simulink model "ModelanfisD1"  (R2017a)
settings: Solver=VariableStepAuto  StartTime=0.0  StopTime=578  RelTol=1e-3
values from neighbouring files (symbols this model uses):
  dinnegc12 = [-0.01 -0.01 -0.02 -0.01 -0.01 -0.01 0 0 0 0 0.01 -0.01 ... (2312 elements, 578x4)]    [anfisd.mat]    (also in anfisfin.mat; cinco.mat)
libraries: dspsrcs4 x84, fuzblock x24
settings Model: Creator=Dell  LastModifiedBy=Dell

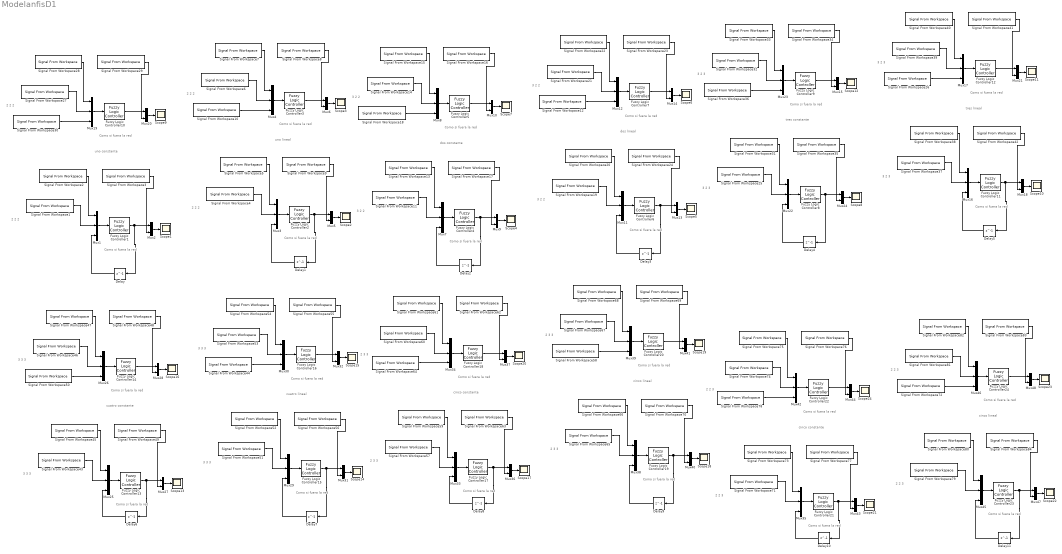
== system ModelanfisD1 ==
  note: 2 2 2
  note: Como si fuera la red
  note: uno constante
  note: 2 2 2
  note: Como si fuera la red
  note: 2 2 2
  note: Como si fuera la red
  note: uno lineal
  note: 2 2 2
  note: Como si fuera la red
  note: 3 2 2
  note: Como si fuera la red
  note: dos constante
  note: 3 2 2
  note: Como si fuera la red
  note: 3 2 2
  note: Como si fuera la red
  note: dos lineal
  note: 3 2 2
  note: Como si fuera la red
  note: 3 2 3
  note: Como si fuera la red
  note: tres constante
  note: 3 2 3
  note: 3 2 3
  note: Como si fuera la red
  note: tres lineal
  note: 3 2 3
  note: Como si fuera la red
  note: 3 3 3
  note: Como si fuera la red
  note: cuatro constante
  note: 3 3 3
  note: Como si fuera la red
  note: 3 3 3
  note: Como si fuera la red
  note: cuatro lineal
  note: 3 3 3
  note: Como si fuera la red
  note: 2 3 3
  note: Como si fuera la red
  note: cinco constante
  note: 2 3 3
  note: Como si fuera la red
  note: 2 3 3
  note: Como si fuera la red
  note: cinco lineal
  note: 2 3 3
  note: Como si fuera la red
  note: 2 2 3
  note: Como si fuera la red
  note: cinco constante
  note: 2 2 3
  note: Como si fuera la red
  note: 2 2 3
  note: Como si fuera la red
  note: cinco lineal
  note: 2 2 3
  note: Como si fuera la red
  Delay{,1..11} (12 alike) : Delay  DelayLength=1  InitialCondition=0
  Fuzzy Logic Controller1 : fuzblock/Fuzzy Logic  Controller  fis=uno
  Fuzzy Logic Controller10 : fuzblock/Fuzzy Logic  Controller  fis=uno
  Fuzzy Logic Controller11 : fuzblock/Fuzzy Logic  Controller  fis=tres3
  Fuzzy Logic Controller12 : fuzblock/Fuzzy Logic  Controller  fis=tres3
  Fuzzy Logic Controller13 : fuzblock/Fuzzy Logic  Controller  fis=cuatro
  Fuzzy Logic Controller14 : fuzblock/Fuzzy Logic  Controller  fis=cuatro
  Fuzzy Logic Controller15 : fuzblock/Fuzzy Logic  Controller  fis=cuatro4
  Fuzzy Logic Controller16 : fuzblock/Fuzzy Logic  Controller  fis=cuatro4
  Fuzzy Logic Controller17 : fuzblock/Fuzzy Logic  Controller  fis=cinco
  Fuzzy Logic Controller18 : fuzblock/Fuzzy Logic  Controller  fis=cinco
  Fuzzy Logic Controller19 : fuzblock/Fuzzy Logic  Controller  fis=cinco5
  Fuzzy Logic Controller2 : fuzblock/Fuzzy Logic  Controller  fis=Uno1
  Fuzzy Logic Controller20 : fuzblock/Fuzzy Logic  Controller  fis=cinco5
  Fuzzy Logic Controller21 : fuzblock/Fuzzy Logic  Controller  fis=seis
  Fuzzy Logic Controller22 : fuzblock/Fuzzy Logic  Controller  fis=seis
  Fuzzy Logic Controller23 : fuzblock/Fuzzy Logic  Controller  fis=seis6
  Fuzzy Logic Controller24 : fuzblock/Fuzzy Logic  Controller  fis=seis6
  Fuzzy Logic Controller3 : fuzblock/Fuzzy Logic  Controller  fis=Uno1
  Fuzzy Logic Controller4 : fuzblock/Fuzzy Logic  Controller  fis=dos
  Fuzzy Logic Controller5 : fuzblock/Fuzzy Logic  Controller  fis=dos
  Fuzzy Logic Controller6 : fuzblock/Fuzzy Logic  Controller  fis=dos2
  Fuzzy Logic Controller7 : fuzblock/Fuzzy Logic  Controller  fis=dos2
  Fuzzy Logic Controller8 : fuzblock/Fuzzy Logic  Controller  fis=tres
  Fuzzy Logic Controller9 : fuzblock/Fuzzy Logic  Controller  fis=tres
  Mux{1,3..4,7..8,11..12,16..17,19,22..23,25..26,29..30,33..35,38..39,42,45..46} (24 alike) : Mux  Inputs=3
  Mux{2,5..6,9..10,13..15,18,20..21,24,27..28,31..32,36..37,40..41,43..44,47..48} (24 alike) : Mux  Inputs=2
  Scope{1..24} (24 alike) : Scope
  Signal From Workspace{1,4,6,11,14,19,21,25,27,32,37,39,43,46,51,53,57,60,65,67,71,74,79,81} (24 alike) : dspsrcs4/Signal From Workspace  X=dinnegc12(:,2)  Ts=1  nsamps=1  OutputAfterFinalValue=Setting to zero  ignoreOrWarnInputAndFrameLengths=off  OutputFrames=off
  Signal From Workspace{10,12,18,26,30,36,44,50,58,64,72,78} (12 alike) : dspsrcs4/Signal From Workspace  X=dinnegc12(:,3)  Ts=1  nsamps=1  OutputAfterFinalValue=Setting to zero  ignoreOrWarnInputAndFrameLengths=off  OutputFrames=off
  Signal From Workspace{2,5,7,13,15,20,22,28,31,33,38,40,45,47,52,54,59,61,66,68,73,75,80,82} (24 alike) : dspsrcs4/Signal From Workspace  X=dinnegc12(:,1)  Ts=1  nsamps=1  OutputAfterFinalValue=Setting to zero  ignoreOrWarnInputAndFrameLengths=off  OutputFrames=off
  Signal From Workspace{3,8..9,16..17,23..24,29,34..35,41..42,48..49,55..56,62..63,69..70,76..77,83..84} (24 alike) : dspsrcs4/Signal From Workspace  X=dinnegc12(:,4)  Ts=1  nsamps=1  OutputAfterFinalValue=Setting to zero  ignoreOrWarnInputAndFrameLengths=off  OutputFrames=off
  wires:
  Signal From Workspace30/1 -> Mux19/3
  Signal From Workspace27/1 -> Mux19/2
  Fuzzy Logic Controller10/1 -> Mux20/1
  Signal From Workspace28/1 -> Mux19/1
  Mux20/1 -> Scope9/1
  Signal From Workspace29/1 -> Mux20/2
  Mux19/1 -> Fuzzy Logic Controller10/1
  Mux1/1 -> Fuzzy Logic Controller1/1
  Signal From Workspace3/1 -> Mux2/2
  Mux2/1 -> Scope1/1
  Signal From Workspace2/1 -> Mux1/1
  Fuzzy Logic Controller1/1 -> Delay/1, Mux2/1
  Signal From Workspace1/1 -> Mux1/2
  Delay/1 -> Mux1/3
  Delay1/1 -> Mux3/3
  Signal From Workspace4/1 -> Mux3/2
  Fuzzy Logic Controller2/1 -> Mux5/1, Delay1/1
  Signal From Workspace5/1 -> Mux3/1
  Mux5/1 -> Scope2/1
  Signal From Workspace9/1 -> Mux5/2
  Mux3/1 -> Fuzzy Logic Controller2/1
  Mux4/1 -> Fuzzy Logic Controller3/1
  Signal From Workspace8/1 -> Mux6/2
  Mux6/1 -> Scope3/1
  Signal From Workspace7/1 -> Mux4/1
  Fuzzy Logic Controller3/1 -> Mux6/1
  Signal From Workspace6/1 -> Mux4/2
  Signal From Workspace10/1 -> Mux4/3
  Signal From Workspace12/1 -> Mux12/3
  Signal From Workspace21/1 -> Mux12/2
  Fuzzy Logic Controller7/1 -> Mux14/1
  Signal From Workspace22/1 -> Mux12/1
  Mux14/1 -> Scope6/1
  Signal From Workspace23/1 -> Mux14/2
  Mux12/1 -> Fuzzy Logic Controller7/1
  Mux11/1 -> Fuzzy Logic Controller6/1
  Signal From Workspace24/1 -> Mux13/2
  Mux13/1 -> Scope5/1
  Signal From Workspace20/1 -> Mux11/1
  Fuzzy Logic Controller6/1 -> Delay3/1, Mux13/1
  Signal From Workspace19/1 -> Mux11/2
  Delay3/1 -> Mux11/3
  Delay2/1 -> Mux7/3
  Signal From Workspace11/1 -> Mux7/2
  Fuzzy Logic Controller4/1 -> Mux9/1, Delay2/1
  Signal From Workspace13/1 -> Mux7/1
  Mux9/1 -> Scope4/1
  Signal From Workspace17/1 -> Mux9/2
  Mux7/1 -> Fuzzy Logic Controller4/1
  Mux8/1 -> Fuzzy Logic Controller5/1
  Signal From Workspace16/1 -> Mux10/2
  Mux10/1 -> Scope7/1
  Signal From Workspace15/1 -> Mux8/1
  Fuzzy Logic Controller5/1 -> Mux10/1
  Signal From Workspace14/1 -> Mux8/2
  Signal From Workspace18/1 -> Mux8/3
  Signal From Workspace36/1 -> Mux23/3
  Signal From Workspace32/1 -> Mux23/2
  Fuzzy Logic Controller9/1 -> Mux15/1
  Signal From Workspace33/1 -> Mux23/1
  Mux15/1 -> Scope12/1
  Signal From Workspace34/1 -> Mux15/2
  Mux23/1 -> Fuzzy Logic Controller9/1
  Mux22/1 -> Fuzzy Logic Controller8/1
  Signal From Workspace35/1 -> Mux24/2
  Mux24/1 -> Scope8/1
  Signal From Workspace31/1 -> Mux22/1
  Fuzzy Logic Controller8/1 -> Delay4/1, Mux24/1
  Signal From Workspace25/1 -> Mux22/2
  Delay4/1 -> Mux22/3
  Delay5/1 -> Mux16/3
  Signal From Workspace37/1 -> Mux16/2
  Fuzzy Logic Controller11/1 -> Delay5/1, Mux18/1
  Signal From Workspace38/1 -> Mux16/1
  Mux18/1 -> Scope10/1
  Signal From Workspace42/1 -> Mux18/2
  Mux16/1 -> Fuzzy Logic Controller11/1
  Mux17/1 -> Fuzzy Logic Controller12/1
  Signal From Workspace41/1 -> Mux21/2
  Mux21/1 -> Scope11/1
  Signal From Workspace40/1 -> Mux17/1
  Fuzzy Logic Controller12/1 -> Mux21/1
  Signal From Workspace39/1 -> Mux17/2
  Signal From Workspace26/1 -> Mux17/3
  Signal From Workspace44/1 -> Mux30/3
  Signal From Workspace53/1 -> Mux30/2
  Fuzzy Logic Controller16/1 -> Mux32/1
  Signal From Workspace54/1 -> Mux30/1
  Mux32/1 -> Scope15/1
  Signal From Workspace55/1 -> Mux32/2
  Mux30/1 -> Fuzzy Logic Controller16/1
  Mux29/1 -> Fuzzy Logic Controller15/1
  Signal From Workspace56/1 -> Mux31/2
  Mux31/1 -> Scope14/1
  Signal From Workspace52/1 -> Mux29/1
  Fuzzy Logic Controller15/1 -> Delay7/1, Mux31/1
  Signal From Workspace51/1 -> Mux29/2
  Delay7/1 -> Mux29/3
  Delay6/1 -> Mux25/3
  Signal From Workspace43/1 -> Mux25/2
  Fuzzy Logic Controller13/1 -> Mux27/1, Delay6/1
  Signal From Workspace45/1 -> Mux25/1
  Mux27/1 -> Scope13/1
  Signal From Workspace49/1 -> Mux27/2
  Mux25/1 -> Fuzzy Logic Controller13/1
  Mux26/1 -> Fuzzy Logic Controller14/1
  Signal From Workspace48/1 -> Mux28/2
  Mux28/1 -> Scope16/1
  Signal From Workspace47/1 -> Mux26/1
  Fuzzy Logic Controller14/1 -> Mux28/1
  Signal From Workspace46/1 -> Mux26/2
  Signal From Workspace50/1 -> Mux26/3
  Signal From Workspace64/1 -> Mux34/3
  Signal From Workspace60/1 -> Mux34/2
  Fuzzy Logic Controller18/1 -> Mux37/1
  Signal From Workspace61/1 -> Mux34/1
  Mux37/1 -> Scope20/1
  Signal From Workspace62/1 -> Mux37/2
  Mux34/1 -> Fuzzy Logic Controller18/1
  Mux33/1 -> Fuzzy Logic Controller17/1
  Signal From Workspace63/1 -> Mux36/2
  Mux36/1 -> Scope17/1
  Signal From Workspace59/1 -> Mux33/1
  Fuzzy Logic Controller17/1 -> Delay8/1, Mux36/1
  Signal From Workspace57/1 -> Mux33/2
  Delay8/1 -> Mux33/3
  Delay9/1 -> Mux38/3
  Signal From Workspace65/1 -> Mux38/2
  Fuzzy Logic Controller19/1 -> Mux40/1, Delay9/1
  Signal From Workspace66/1 -> Mux38/1
  Mux40/1 -> Scope18/1
  Signal From Workspace70/1 -> Mux40/2
  Mux38/1 -> Fuzzy Logic Controller19/1
  Mux39/1 -> Fuzzy Logic Controller20/1
  Signal From Workspace69/1 -> Mux41/2
  Mux41/1 -> Scope19/1
  Signal From Workspace68/1 -> Mux39/1
  Fuzzy Logic Controller20/1 -> Mux41/1
  Signal From Workspace67/1 -> Mux39/2
  Signal From Workspace58/1 -> Mux39/3
  Signal From Workspace72/1 -> Mux46/3
  Signal From Workspace81/1 -> Mux46/2
  Fuzzy Logic Controller24/1 -> Mux48/1
  Signal From Workspace82/1 -> Mux46/1
  Mux48/1 -> Scope23/1
  Signal From Workspace83/1 -> Mux48/2
  Mux46/1 -> Fuzzy Logic Controller24/1
  Mux45/1 -> Fuzzy Logic Controller23/1
  Signal From Workspace84/1 -> Mux47/2
  Mux47/1 -> Scope22/1
  Signal From Workspace80/1 -> Mux45/1
  Fuzzy Logic Controller23/1 -> Delay11/1, Mux47/1
  Signal From Workspace79/1 -> Mux45/2
  Delay11/1 -> Mux45/3
  Delay10/1 -> Mux35/3
  Signal From Workspace71/1 -> Mux35/2
  Fuzzy Logic Controller21/1 -> Mux43/1, Delay10/1
  Signal From Workspace73/1 -> Mux35/1
  Mux43/1 -> Scope21/1
  Signal From Workspace77/1 -> Mux43/2
  Mux35/1 -> Fuzzy Logic Controller21/1
  Mux42/1 -> Fuzzy Logic Controller22/1
  Signal From Workspace76/1 -> Mux44/2
  Mux44/1 -> Scope24/1
  Signal From Workspace75/1 -> Mux42/1
  Fuzzy Logic Controller22/1 -> Mux44/1
  Signal From Workspace74/1 -> Mux42/2
  Signal From Workspace78/1 -> Mux42/3
